simulink model "sus2"  (R2018a)
settings: Solver=ode23t  StartTime=0.0  StopTime=2.5  EnableMultiTasking=on
PreLoadFcn:
  | load carParams
values from neighbouring files (symbols this model uses):
  b1 = 25    [matlab2.mat]
  b2 = 0    [matlab2.mat]
  b3 = 1000    [matlab2.mat]
  b4 = 0    [matlab2.mat]
  k1 = 8100    [matlab2.mat]
  k2 = 23000    [matlab2.mat]
  k3 = 60000    [matlab2.mat]
  k4 = 60000    [matlab2.mat]
  mCarF = 100    [matlab2.mat]
  mCarR = 150    [matlab2.mat]
  mWheelF = 12    [matlab2.mat]
  mWheelR = 16    [matlab2.mat]
settings Model: Creator=scastro  LastModifiedBy=Prana
settings DataIOCC: SaveFormat=Array  OutputTimes=0:0.001:60
settings OptimizationCC: LifeSpan=inf
settings DebuggingCC: SFUnexpectedBacktrackingDiag=warning  SFNoUnconditionalDefaultTransitionDiag=warning  SFExecutionAtInitializationDiag=none
settings HardwareCC: ProdBitPerPointer=32  ProdBitPerSizeT=32  ProdBitPerPtrDiffT=32  ProdLargestAtomicFloat=None  ProdIntDivRoundTo=Undefined  ProdEndianess=Unspecified  ProdWordSize=32  ProdHWDeviceType=32-bit Generic
settings ModelReferenceCC: PropagateSignalLabelsOutOfModel=off
settings CodeAppCC: StateflowObjectComments=on
settings GRTTargetCC: TargetLangStandard=C89/C90 (ANSI)  GeneratePreprocessorConditionals=Disable all
settings ConfigComp: CovMetricSettings=dw  CovHtmlReporting=on  CovSaveCumulativeToWorkspaceVar=on  CovSaveSingleToWorkspaceVar=on  CovExternalEMLEnable=off
settings SimscapeCC: SimscapeNormalizeSystem=off  SimscapeLogType=all  SimscapeLogDataHistory=10000
settings ConfigurationSet: Description=SimMechanics 2G

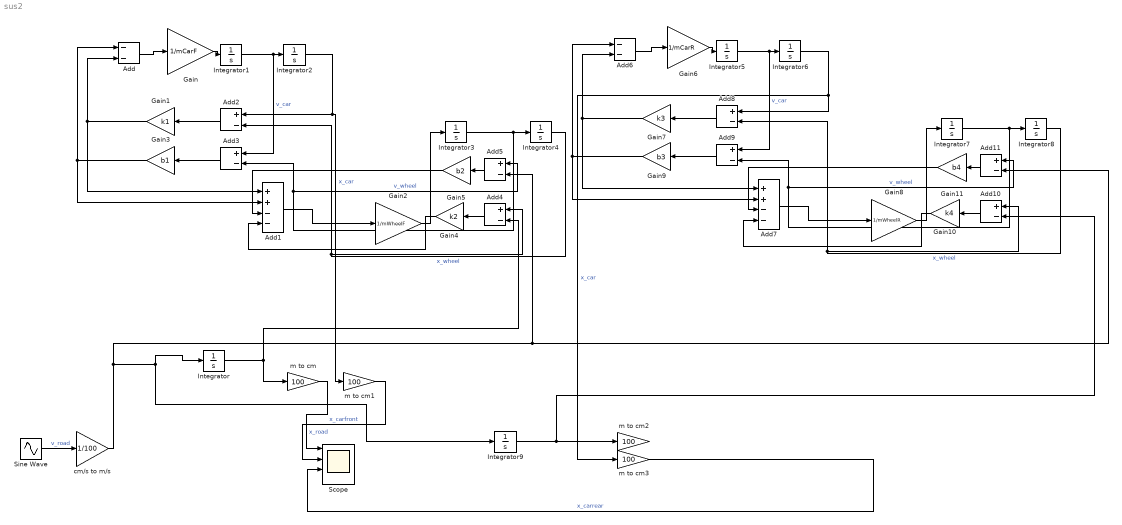
== system sus2 ==
  Add : Sum  Inputs=--
  Add1 : Sum  Inputs=++--
  Add{2..5,8..11} (8 alike) : Sum  Inputs=+-
  Add6 : Sum  Inputs=--
  Add7 : Sum  Inputs=++--
  Gain : Gain  Gain=1/mCarF
  Gain1 : Gain  Gain=k1
  Gain10 : Gain  Gain=k4
  Gain11 : Gain  Gain=b4
  Gain2 : Gain  Gain=1/mWheelF
  Gain3 : Gain  Gain=b1
  Gain4 : Gain  Gain=k2
  Gain5 : Gain  Gain=b2
  Gain6 : Gain  Gain=1/mCarR
  Gain7 : Gain  Gain=k3
  Gain8 : Gain  Gain=1/mWheelR
  Gain9 : Gain  Gain=b3
  Integrator{,1..9} (10 alike) : Integrator
  Scope : Scope  NumInputPorts=4
  Sine Wave : Sin  Amplitude=4500  Frequency=300  Phase=pi/2  SampleTime=0
  cm/s to m/s : Gain  Gain=1/100
  m to cm{,1..3} (4 alike) : Gain  Gain=100
  wires:
  Integrator/1 -> Add4/2, m to cm/1
  Gain/1 -> Integrator1/1
  Add/1 -> Gain/1
  Integrator2/1 -> Add2/1, m to cm1/1  "x_car"
  Integrator1/1 -> Add3/1, Integrator2/1  "v_car"
  Gain2/1 -> Integrator3/1
  Add1/1 -> Gain2/1
  Integrator4/1 -> Add2/2, Add4/1  "x_wheel"
  Integrator3/1 -> Add3/2, Add5/1, Integrator4/1  "v_wheel"
  Add2/1 -> Gain1/1
  Add3/1 -> Gain3/1
  Gain1/1 -> Add1/1, Add/2
  Gain3/1 -> Add1/2, Add/1
  Add4/1 -> Gain4/1
  Gain4/1 -> Add1/4
  Add5/1 -> Gain5/1
  Gain5/1 -> Add1/3
  Sine Wave/1 -> cm/s to m/s/1  "v_road"
  m to cm/1 -> Scope/1  "x_road"
  m to cm1/1 -> Scope/2  "x_carfront"
  Integrator7/1 -> Add9/2, Add11/1, Integrator8/1  "v_wheel"
  Gain11/1 -> Add7/3
  Integrator8/1 -> Add8/2, Add10/1  "x_wheel"
  Gain10/1 -> Add7/4
  Integrator5/1 -> Add9/1, Integrator6/1  "v_car"
  Add8/1 -> Gain7/1
  Gain9/1 -> Add7/2, Add6/1
  Gain7/1 -> Add7/1, Add6/2
  Add7/1 -> Gain8/1
  Add9/1 -> Gain9/1
  Add10/1 -> Gain10/1
  Gain8/1 -> Integrator7/1
  Add11/1 -> Gain11/1
  Integrator6/1 -> Add8/1, m to cm3/1  "x_car"
  Integrator9/1 -> Add10/2, m to cm2/1
  Gain6/1 -> Integrator5/1
  Add6/1 -> Gain6/1
  cm/s to m/s/1 -> Add11/2, Add5/2, Integrator9/1, Integrator/1
  m to cm3/1 -> Scope/3  "x_carrear"
